simulink model "PI_controller"  (R2023a)
settings: Solver=VariableStepAuto  StartTime=0.0  StopTime=1500  RelTol=1e-3
values from neighbouring files (symbols this model uses):
  A = 332.5    [initializare_model.m]
  ho = 17.38    [initializare_model.m]
  hss = 20.86    [initializare_model.m]
  k = 0.033    [initializare_model.m]
  k11 = k2^2 + 4*(k - k3)*k1    (= 0.0881226)    [initializare_model.m]
  k12 = 8*(k - k3)    (= 0.2688)    [initializare_model.m]
  k13 = 2*(k - k3)    (= 0.0672)    [initializare_model.m]
  k2 = -0.015    [initializare_model.m]
  keta = 8e-5    (= 8e-05)    [initializare_model.m]
  Kp = h/u    (= 2.32)    [initializare_model.m]
  qo = 37.63    [initializare_model.m]
  Tp = 225    [initializare_model.m]
libraries: slpidlib x1
settings Model: Creator=evely  LastModifiedBy=evely

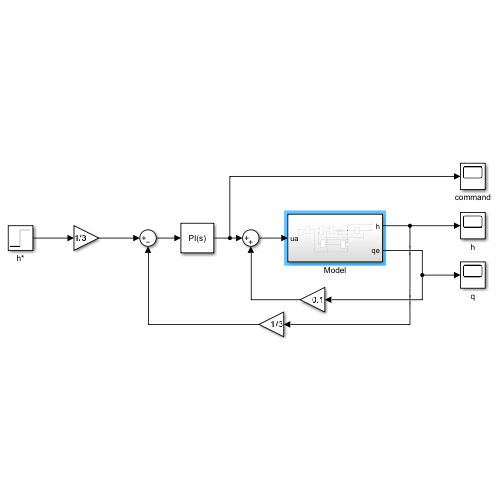
[thumbnail: Simulink's stored preview of the top-level diagram]
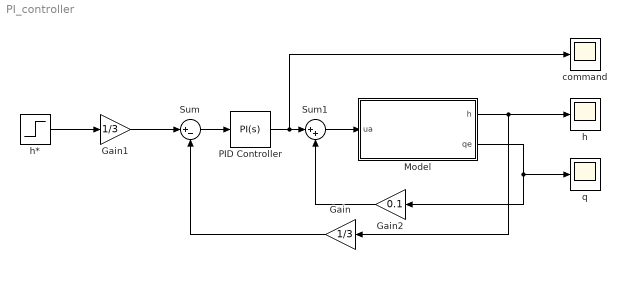
== system PI_controller ==
  Gain : Gain  Gain=1/3
  Gain1 : Gain  Gain=1/3
  Gain2 : Gain  Gain=0.1
  Model : Subsystem
  PID Controller : slpidlib/PID Controller  Controller=PI  Form=Ideal  TimeDomain=Continuous-time  UseExternalTs=off  SampleTime=-1  IntegratorMethod=Forward Euler  FilterMethod=Forward Euler  ControllerParametersSource=internal  P=Kp  I=1/Tp  UseKiTs=off  D=0  N=100  UseFilter=on  TunerSelectOption=Transfer Function Based (PID Tuner App)  InitialConditionSource=internal  InitialConditionForIntegrator=4.4  InitialConditionForFilter=0  DifferentiatorICPrevScaledInput=0  ExternalReset=none  TrackingMode=off  Kt=1  LimitOutput=off  SatLimitsSource=internal  UpperSaturationLimit=inf  LowerSaturationLimit=-inf  LinearizeAsGain=on  AntiWindupMode=none  Kb=1  LimitIntegrator=off  UpperIntegratorSaturationLimit=inf  LowerIntegratorSaturationLimit=-inf  POutMin=[]  POutMax=[]  IOutMin=[]  IOutMax=[]  DOutMin=[]  DOutMax=[]  NOutMin=[]  NOutMax=[]  SumOutMin=[]  SumOutMax=[]  SaturationOutMin=[]  SaturationOutMax=[]  PParamMin=[]  PParamMax=[]  IParamMin=[]  IParamMax=[]  DParamMin=[]  DParamMax=[]  NParamMin=[]  NParamMax=[]  KbParamMin=[]  KbParamMax=[]  KtParamMin=[]  KtParamMax=[]  KbOutMin=[]  KbOutMax=[]  KtOutMin=[]  KtOutMax=[]  IntegratorOutMin=[]  IntegratorOutMax=[]  FilterOutMin=[]  FilterOutMax=[]  SumI1OutMin=[]  SumI1OutMax=[]  SumI2OutMin=[]  SumI2OutMax=[]  SumI3OutMin=[]  SumI3OutMax=[]  SumI4OutMin=[]  SumI4OutMax=[]  SumDOutMin=[]  SumDOutMax=[]  DifferentiatorOutMin=[]  DifferentiatorOutMax=[]  FilterDiffOutCoefMin=[]  FilterDiffOutCoefMax=[]  ReciprocalOutMin=[]  ReciprocalOutMax=[]  SumDenOutMin=[]  SumDenOutMax=[]  SumNumOutMin=[]  SumNumOutMax=[]  DivideOutMin=[]  DivideOutMax=[]  UdiffTsProdOutMin=[]  UdiffTsProdOutMax=[]  NTsProdOutMin=[]  NTsProdOutMax=[]  UintegralTsProdOutMin=[]  UintegralTsProdOutMax=[]  UngainTsProdOutMin=[]  UngainTsProdOutMax=[]  ClampingZeroOutDataTypeStr=Inherit: Inherit via back propagation  ClampingZeroOutMin=[]  ClampingZeroOutMax=[]  FilterDenConstantOutDataTypeStr=Inherit: Inherit via back propagation  FilterDenConstantOutMin=[]  FilterDenConstantOutMax=[]  PCopyOutDataTypeStr=Inherit: Inherit via back propagation  PCopyOutMin=[]  PCopyOutMax=[]  NCopyOutDataTypeStr=Inherit: Inherit via back propagation  NCopyOutMin=[]  NCopyOutMax=[]  IntegratorContinuousStateAttributes=''  IntegratorStateMustResolveToSignalObject=off  IntegratorRTWStateStorageClass=Auto  FilterContinuousStateAttributes=''  FilterStateMustResolveToSignalObject=off  FilterRTWStateStorageClass=Auto  ParallelPVariant=Passthrough  IdealPVariant=InternalParameters  IVariant=InternalParameters  DVariant=Disabled  IntegratorVariant=Continuous  SatVariant=Disabled  AWVariant=Passthrough  PCopyVariant=Disabled  TRVariant=Disabled  FdbkBlocksVariant=Forward  IdealPFdbkVariant=Disabled  SatFdbkVariant=Disabled  DerivativeFilterVariant=Disabled  NVariant=Disabled  NCopyVariant=Disabled_SignalSpec  FilterICVariant=Disabled  IntegratorICVariant=InternalICs  ExternalResetVariant=Disabled  TRSumVariant=Passthrough  SumFdbkVariant=Disabled  SumVariant=Sum_PI  TsampFilterVariant=InternalTs  TsampNgainVariant=Passthrough  TsampIntegralVariant=Disabled_SignalSpec  ExternalSaturationOutDataTypeStr=Inherit: Same as second input
  Sum : Sum  Inputs=|+-
  Sum1 : Sum  Inputs=|++
  command : Scope
  h : Scope
  h* : Step  Time=0  Before=ho  After=hss  SampleTime=0
  q : Scope
  wires:
  Gain/1 -> Sum/2
  Sum1/1 -> Model/1(ua)
  Sum/1 -> PID Controller/1
  Gain2/1 -> Sum1/2
  Gain1/1 -> Sum/1
  h*/1 -> Gain1/1
  PID Controller/1 -> Sum1/1, command/1
  Model/2(qe) -> Gain2/1, q/1
  Model/1(h) -> Gain/1, h/1

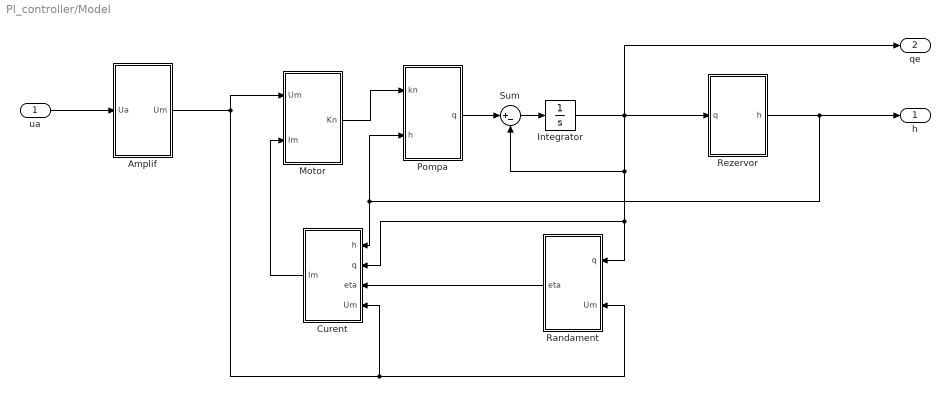
== system PI_controller/Model ==
  ua : Inport
  Amplif : Subsystem
  Curent : Subsystem
  Integrator : Integrator  InitialCondition=qo
  Motor : Subsystem
  Pompa : Subsystem
  Randament : Subsystem
  Rezervor : Subsystem
  Sum : Sum  Inputs=|+-
  h : Outport
  qe : Outport  Port=2
  wires:
  ua/1 -> Amplif/1(Ua)
  Sum/1 -> Integrator/1
  Integrator/1 -> Sum/2, Randament/1(q), Curent/2(q), Rezervor/1(q), qe/1
  Rezervor/1(h) -> Pompa/2(h), Curent/1(h), h/1
  Amplif/1(Um) -> Motor/1(Um), Randament/2(Um), Curent/4(Um)
  Motor/1(Kn) -> Pompa/1(kn)
  Randament/1(eta) -> Curent/3(eta)
  Curent/1(Im) -> Motor/2(Im)
  Pompa/1(q) -> Sum/1

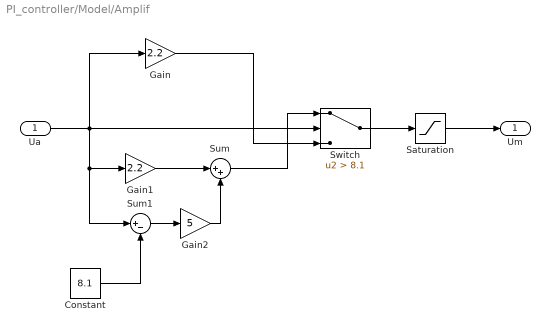
== system PI_controller/Model/Amplif ==
  Ua : Inport
  Constant : Constant  Value=8.1
  Gain : Gain  Gain=2.2
  Gain1 : Gain  Gain=2.2
  Gain2 : Gain  Gain=5
  Saturation : Saturate  UpperLimit=22  LowerLimit=0
  Sum : Sum  Inputs=|++
  Sum1 : Sum  Inputs=|+-
  Switch : Switch  Criteria=u2 > Threshold  Threshold=8.1  SaturateOnIntegerOverflow=off  InputSameDT=off
  Um : Outport
  wires:
  Ua/1 -> Gain1/1, Sum1/1, Gain/1, Switch/2
  Gain/1 -> Switch/3
  Switch/1 -> Saturation/1
  Gain1/1 -> Sum/1
  Constant/1 -> Sum1/2
  Sum1/1 -> Gain2/1
  Gain2/1 -> Sum/2
  Sum/1 -> Switch/1
  Saturation/1 -> Um/1

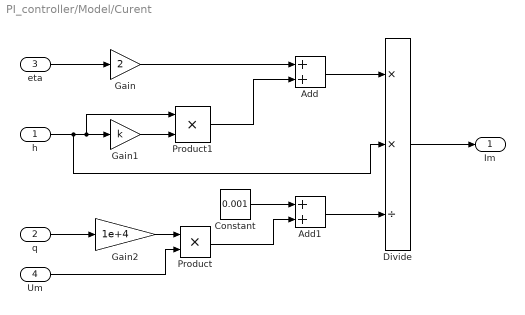
== system PI_controller/Model/Curent ==
  h : Inport
  q : Inport  Port=2
  eta : Inport  Port=3
  Um : Inport  Port=4
  Add : Sum
  Add1 : Sum
  Constant : Constant  Value=0.001
  Divide : Product  Inputs=**/
  Gain : Gain  Gain=2
  Gain1 : Gain  Gain=k
  Gain2 : Gain  Gain=1e+4
  Product : Product
  Product1 : Product
  Im : Outport
  wires:
  eta/1 -> Gain/1
  Gain/1 -> Add/1
  h/1 -> Divide/2, Product1/1, Gain1/1
  Gain1/1 -> Product1/2
  Add/1 -> Divide/1
  Product1/1 -> Add/2
  Divide/1 -> Im/1
  q/1 -> Gain2/1
  Gain2/1 -> Product/1
  Um/1 -> Product/2
  Constant/1 -> Add1/1
  Product/1 -> Add1/2
  Add1/1 -> Divide/3

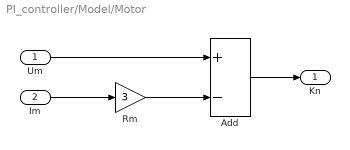
== system PI_controller/Model/Motor ==
  Um : Inport
  Im : Inport  Port=2
  Add : Sum  Inputs=+-
  Rm : Gain  Gain=3
  Kn : Outport
  wires:
  Im/1 -> Rm/1
  Rm/1 -> Add/2
  Um/1 -> Add/1
  Add/1 -> Kn/1

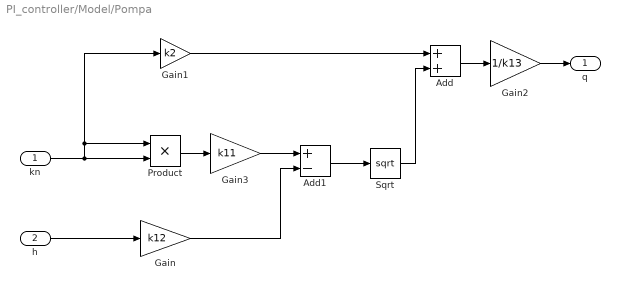
== system PI_controller/Model/Pompa ==
  kn : Inport
  h : Inport  Port=2
  Add : Sum
  Add1 : Sum  Inputs=+-
  Gain : Gain  Gain=k12
  Gain1 : Gain  Gain=k2
  Gain2 : Gain  Gain=1/k13
  Gain3 : Gain  Gain=k11
  Product : Product
  Sqrt : Sqrt
  q : Outport
  wires:
  kn/1 -> Product/1, Gain1/1, Product/2
  Gain1/1 -> Add/1
  Add/1 -> Gain2/1
  Gain2/1 -> q/1
  h/1 -> Gain/1
  Product/1 -> Gain3/1
  Gain3/1 -> Add1/1
  Add1/1 -> Sqrt/1
  Gain/1 -> Add1/2
  Sqrt/1 -> Add/2

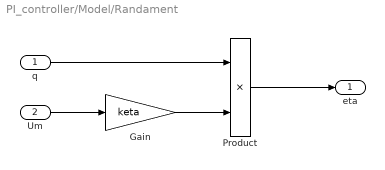
== system PI_controller/Model/Randament ==
  q : Inport
  Um : Inport  Port=2
  Gain : Gain  Gain=keta
  Product : Product
  eta : Outport
  wires:
  q/1 -> Product/1
  Product/1 -> eta/1
  Um/1 -> Gain/1
  Gain/1 -> Product/2

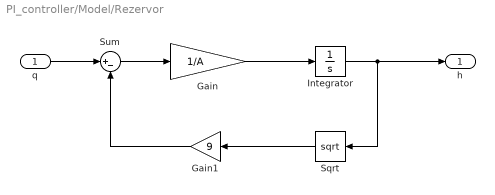
== system PI_controller/Model/Rezervor ==
  q : Inport
  Gain : Gain  Gain=1/A
  Gain1 : Gain  Gain=9
  Integrator : Integrator  InitialCondition=ho
  Sqrt : Sqrt
  Sum : Sum  Inputs=|+-
  h : Outport
  wires:
  q/1 -> Sum/1
  Sum/1 -> Gain/1
  Gain/1 -> Integrator/1
  Integrator/1 -> Sqrt/1, h/1
  Sqrt/1 -> Gain1/1
  Gain1/1 -> Sum/2
